simulink model "non_linear_system"  (R2021b)
settings: Solver=VariableStepAuto  StartTime=0.0  StopTime=10.0  RelTol=1e-3
settings Model: Creator=Anubhav Paras  LastModifiedBy=vanshika
settings SolverCC: AlgebraicLoopSolver=TrustRegion
settings DebuggingCC: SFMachineParentedDataDiag=warning

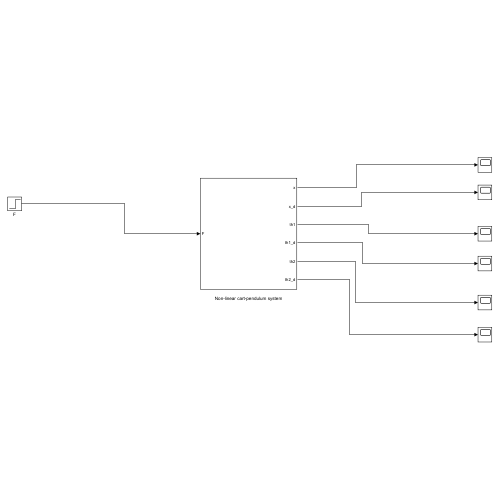
[thumbnail: Simulink's stored preview of the top-level diagram]
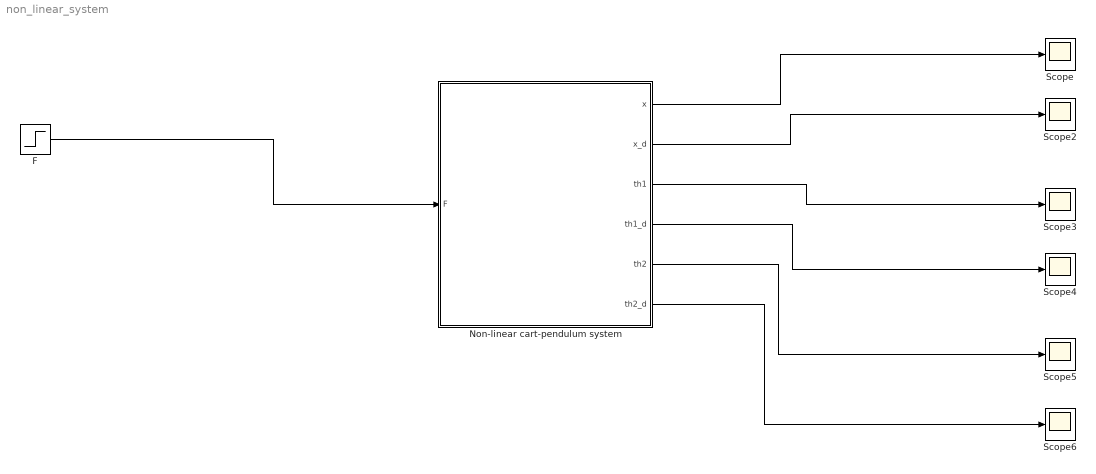
== system non_linear_system ==
  " Non-linear cart-pendulum system" : Subsystem
  F : Step  SampleTime=0
  Scope{,2..6} (6 alike) : Scope
  wires:
  F/1 -> " Non-linear cart-pendulum system"/1(F)
  " Non-linear cart-pendulum system"/1(x) -> Scope/1
  " Non-linear cart-pendulum system"/2(x_d) -> Scope2/1
  " Non-linear cart-pendulum system"/3(th1) -> Scope3/1
  " Non-linear cart-pendulum system"/4(th1_d) -> Scope4/1
  " Non-linear cart-pendulum system"/5(th2) -> Scope5/1
  " Non-linear cart-pendulum system"/6(th2_d) -> Scope6/1

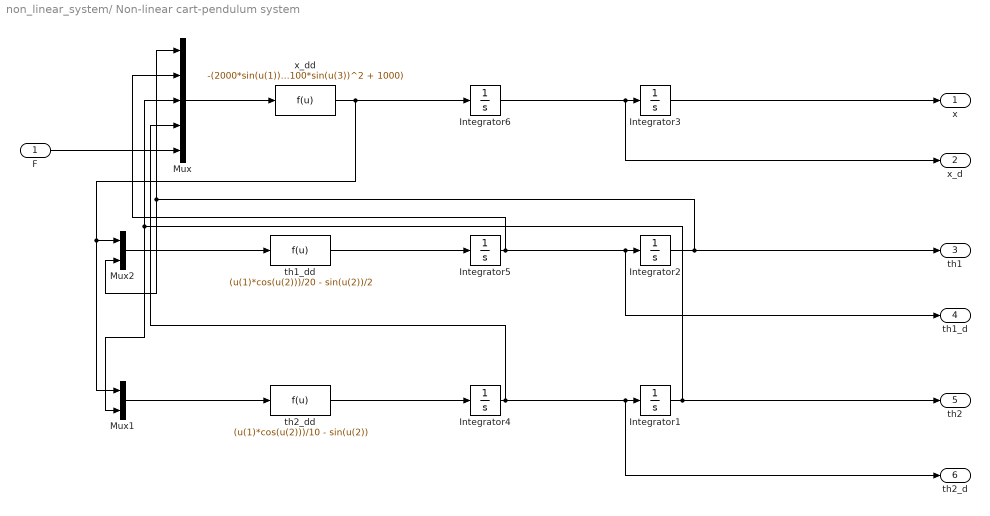
== system non_linear_system/ Non-linear cart-pendulum system ==
  F : Inport
  Integrator{1..6} (6 alike) : Integrator
  Mux : Mux  Inputs=5
  Mux1 : Mux  Inputs=2
  Mux2 : Mux  Inputs=2
  th1_dd : Fcn  Expr=(u(1)*cos(u(2)))/20 - sin(u(2))/2
  th2_dd : Fcn  Expr=(u(1)*cos(u(2)))/10 - sin(u(2))
  x_dd : Fcn  Expr=-(2000*sin(u(1))*u(2)^2 + 1000*sin(u(3))*u(4)^2 - u(5) + 1000*cos(u(1))*sin(u(1)) - 1000*cos(u(3))*sin(u(3)))/(100*sin(u(1))^2 + 100*sin(u(3))^2 + 1000)
  x : Outport
  x_d : Outport  Port=2
  th1 : Outport  Port=3
  th1_d : Outport  Port=4
  th2 : Outport  Port=5
  th2_d : Outport  Port=6
  wires:
  th2_dd/1 -> Integrator4/1
  x_dd/1 -> Mux1/1, Mux2/1, Integrator6/1
  Integrator6/1 -> x_d/1, Integrator3/1
  Mux1/1 -> th2_dd/1
  Integrator5/1 -> Mux/2, th1_d/1, Integrator2/1
  Mux/1 -> x_dd/1
  Integrator1/1 -> th2/1, Mux1/2, Mux/3
  Integrator2/1 -> th1/1, Mux2/2, Mux/1
  th1_dd/1 -> Integrator5/1
  Integrator4/1 -> Mux/4, th2_d/1, Integrator1/1
  Mux2/1 -> th1_dd/1
  Integrator3/1 -> x/1
  F/1 -> Mux/5
